simulink model "reverbe1"  (R2019a)
settings: Solver=VariableStepAuto  StartTime=0.0  StopTime=30  RelTol=1e-3
libraries: dspvision x1, dspobslib x1, Librairie x1
settings Model: Creator=shse  LastModifiedBy=shse

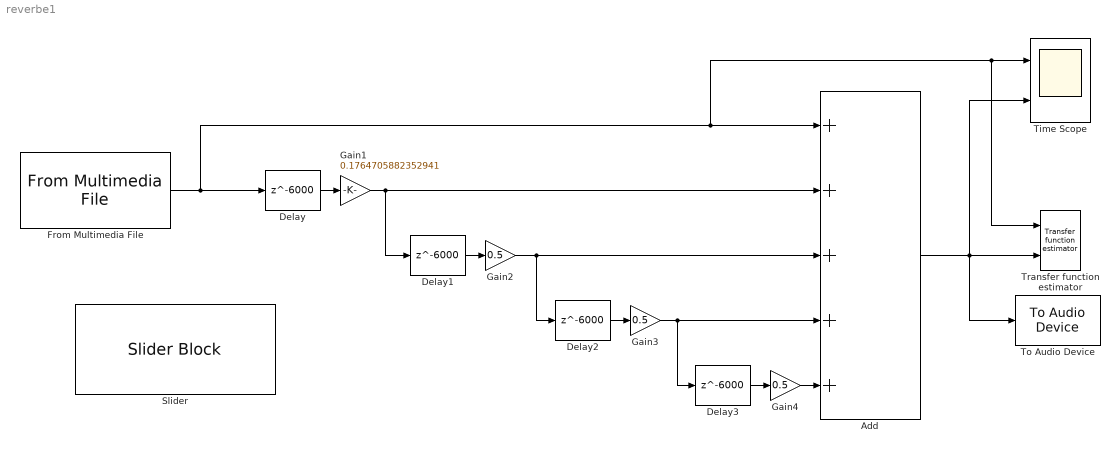
== system reverbe1 ==
  Add : Sum  Inputs=+++++
  Delay{,1..3} (4 alike) : Delay  DelayLength=6000  DelayLengthUpperLimit=5000  InputProcessing=Columns as channels (frame based)
  From Multimedia File : dspvision/From Multimedia File  inputFilename=C:\Users\shse\Nextcloud\L3\LU3EE105\Audio\Documents de TP et projet-20191118\Projet\batterie.wav  readRange=[1 Inf]  loop=on  numPlays=inf  outputStreams=Audio only  videoDataType=single  audioDataType=double  inheritSampleTime=on  userDefinedSampleTime=1/30  noAudioOutput=off  isIntensityVideo=off  fourcc=RGB  colorVideoFormat=Separate color signals  outputEOF=off  dataOrg=Column-major  audioFrameSize=1024  computeAudioFrameSize=off  outSamplingMode=Sample based
      settings: SourceProductName=DSP System Toolbox  SourceProductBaseCode=DS
  Gain1 : Gain  Gain=0.1764705882352941
  Gain2 : Gain  Gain=0.5
  Gain3 : Gain  Gain=0.5
  Gain4 : Gain  Gain=0.5
  Slider : SliderBlock  ScaleMax=1
  Time Scope : Scope  NumInputPorts=2
  To Audio Device : dspobslib/To Audio Device  deviceName=Default  inheritSampleRate=on  sampleRate=44100  deviceDatatype=Determine from input data type  autoBufferSize=on  bufferSize=4096  queueDuration=1.0  defaultOutputChannelMapping=on  outputChannelMapping=1:2  outputNumUnderrunSamples=off
      settings: SourceProductName=DSP System Toolbox  SourceProductBaseCode=DS
  Transfer function estimator : Librairie/Transfer function estimator  fee=48000  NN=1024
  wires:
  Delay/1 -> Gain1/1
  Gain1/1 -> Delay1/1, Add/2
  From Multimedia File/1 -> Delay/1, Transfer function estimator/1, Time Scope/1, Add/1
  Add/1 -> To Audio Device/1, Time Scope/2, Transfer function estimator/2
  Delay1/1 -> Gain2/1
  Gain2/1 -> Delay2/1, Add/3
  Delay2/1 -> Gain3/1
  Gain3/1 -> Delay3/1, Add/4
  Delay3/1 -> Gain4/1
  Gain4/1 -> Add/5
